simulink model "SF042A_HwAgSnsrls"  (R2013b)
settings: Solver=FixedStepDiscrete  SolverMode=SingleTasking  StartTime=0.0  StopTime=1  FixedStep=0.002  RelTol=1e-3
values from neighbouring files (symbols this model uses):
  ARCHGLBPRM_2MILLISEC_SEC_F32 = DataDict.Constant    [SF042A_HwAgSnsrls_DataDict.m]
  CORRDPINIONAGCON_CNT_U08 = DataDict.Constant    [SF042A_HwAgSnsrls_DataDict.m]
  FCENTROFFSCON_CNT_U08 = DataDict.Constant    [SF042A_HwAgSnsrls_DataDict.m]
  HwAgSnsrlsCorrdPinionAgHwConf = DataDict.Calibration    [SF042A_HwAgSnsrls_DataDict.m]
  HwAgSnsrlsFCentrHwConf = DataDict.Calibration    [SF042A_HwAgSnsrls_DataDict.m]
  HwAgSnsrlsSmotngCoeff = DataDict.Calibration    [SF042A_HwAgSnsrls_DataDict.m]
  HwAgSnsrlsSmotngStepThd = DataDict.Calibration    [SF042A_HwAgSnsrls_DataDict.m]
  HwAgSnsrlsStordPinionConf = DataDict.Calibration    [SF042A_HwAgSnsrls_DataDict.m]
  HwAgSnsrlsStordPinionConfThd = DataDict.Calibration    [SF042A_HwAgSnsrls_DataDict.m]
  HwAgSnsrlsVehDynDifThd = DataDict.Calibration    [SF042A_HwAgSnsrls_DataDict.m]
  HwAgSnsrlsVehDynHwConf = DataDict.Calibration    [SF042A_HwAgSnsrls_DataDict.m]
  HwAgSnsrlsVehDynMotVelThd = DataDict.Calibration    [SF042A_HwAgSnsrls_DataDict.m]
  HwAgSnsrlsVehDynPinionTqThd = DataDict.Calibration    [SF042A_HwAgSnsrls_DataDict.m]
  HwAgSnsrlsVehDynTmr1Thd = DataDict.Calibration    [SF042A_HwAgSnsrls_DataDict.m]
  HwAgSnsrlsVehDynTmr2Thd = DataDict.Calibration    [SF042A_HwAgSnsrls_DataDict.m]
  HwAgSnsrlsVehDynVehSpdThd = DataDict.Calibration    [SF042A_HwAgSnsrls_DataDict.m]
  HwAgSnsrlsVehDynYawRateThd = DataDict.Calibration    [SF042A_HwAgSnsrls_DataDict.m]
  HwAgSnsrlsWhlFrqThd = DataDict.Calibration    [SF042A_HwAgSnsrls_DataDict.m]
  HwAgSnsrlsWhlSpdHwAgCoeff1 = DataDict.Calibration    [SF042A_HwAgSnsrls_DataDict.m]
  HwAgSnsrlsWhlSpdHwAgCoeff2 = DataDict.Calibration    [SF042A_HwAgSnsrls_DataDict.m]
  HwAgSnsrlsWhlSpdHwAgThd = DataDict.Calibration    [SF042A_HwAgSnsrls_DataDict.m]
  HwAgSnsrlsWhlSpdHwConf = DataDict.Calibration    [SF042A_HwAgSnsrls_DataDict.m]
  HwAgSnsrlsWhlSpdRatThd = DataDict.Calibration    [SF042A_HwAgSnsrls_DataDict.m]
  HwAgSnsrlsWhlSpdTmrThd = DataDict.Calibration    [SF042A_HwAgSnsrls_DataDict.m]
  HwAgSnsrlsWhlSpdVehSpdThd = DataDict.Calibration    [SF042A_HwAgSnsrls_DataDict.m]
  LASTPOSNCON_CNT_U08 = DataDict.Constant    [SF042A_HwAgSnsrls_DataDict.m]
  MILLISECTO100MICROSEC_ULS_U32 = DataDict.Constant    [SF042A_HwAgSnsrls_DataDict.m]
  SysGlbPrmSysKineRat = DataDict.ImprtdCal    [SF042A_HwAgSnsrls_DataDict.m]
  SysGlbPrmSysTqRat = DataDict.ImprtdCal    [SF042A_HwAgSnsrls_DataDict.m]
  VEHDYNCON_CNT_U08 = DataDict.Constant    [SF042A_HwAgSnsrls_DataDict.m]
  WHLSPDCON_CNT_U08 = DataDict.Constant    [SF042A_HwAgSnsrls_DataDict.m]
undefined symbols (not defined in the file or in its folder): NtcNr1, SigQlfr1
libraries: NxtrAbslt x11, Fil x8, NxtrLim x4, simulink x3, NxtrNvM x1, FixdToFloat x1
(part 1 of 6)
settings Model: Creator=BZHF94  LastModifiedBy=bzhf94
settings SolverCC: AutoInsertRateTranBlk=on  InsertRTBMode=Always
settings DataIOCC: LimitDataPoints=off  SaveFormat=Structure  ReturnWorkspaceOutputs=on
settings OptimizationCC: BlockReduction=off  InlineParams=on  ZeroExternalMemoryAtStartup=off  ZeroInternalMemoryAtStartup=off  OptimizeModelRefInitCode=on  LifeSpan=1
settings DebuggingCC: SignalInfNanChecking=error  SignalRangeChecking=warning  UnderspecifiedInitializationDetection=Simplified  SolverPrmCheckMsg=error  InheritedTsInSrcMsg=error  DiscreteInheritContinuousMsg=error  SingleTaskRateTransMsg=error  TasksWithSamePriorityMsg=error  SigSpecEnsureSampleTimeMsg=error  CheckMatrixSingularityMsg=error  ParameterUnderflowMsg=error  ParameterPrecisionLossMsg=error  ParameterTunabilityLossMsg=error  FixptConstUnderflowMsg=warning  FixptConstOverflowMsg=warning  VectorMatrixConversionMsg=error  SignalLabelMismatchMsg=error  UnconnectedInputMsg=error  UnconnectedOutputMsg=error  UnconnectedLineMsg=error  SFcnCompatibilityMsg=error  UniqueDataStoreMsg=warning  BusObjectLabelMismatch=error  RootOutportRequireBusObject=error  AssertControl=DisableAll  ModelReferenceIOMsg=error  ModelReferenceVersionMismatchMessage=warning  ModelReferenceIOMismatchMessage=error  ModelReferenceCSMismatchMessage=warning  ModelReferenceDataLoggingMessage=error  StateNameClashWarn=warning  StrictBusMsg=ErrorOnBusTreatedAsVector  NonBusSignalsTreatedAsBus=error  SFUnexpectedBacktrackingDiag=error  SFInvalidInputDataAccessInChartInitDiag=error  SFNoUnconditionalDefaultTransitionDiag=error  SFTransitionOutsideNaturalParentDiag=error  SFUnconditionalTransitionShadowingDiag=error  SFUndirectedBroadcastEventsDiag=error
settings ModelReferenceCC: ModelReferenceNumInstancesAllowed=Single
settings RTWCC: SystemTargetFile=autosar.tlc  GenCodeOnly=on  TemplateMakefile=ert_default_tmf  Description=AUTOSAR  GenerateReport=on  ProcessScript=autosar_make_rtw_hook  LaunchReport=on
settings CodeAppCC: GenerateComments=off  IgnoreCustomStorageClasses=off  CustomSymbolStrType=$N$R$M  CustomSymbolStrBlkIO=$N$M  SimulinkBlockComments=off
settings STFCustomTargetCC: ParMdlRefBuildCompliant=on  CompOptLevelCompliant=on  IncludeMdlTerminateFcn=off  CombineOutputUpdateFcns=on  SuppressErrorStatus=on  ERTFirstTimeCompliant=on  ERTCustomFileBanners=on  SupportNonFinite=off  SupportComplex=off  SupportContinuousTime=off  SupportNonInlinedSFcns=off  MATLABClassNameForMDSCustomization=Simulink.SoftwareTarget.ERTCustomization  AutosarCompliant=on  GRTInterface=off  SystemTargetFile=autosar.tlc
settings ERTTargetCC: CodeReplacementLibrary=ANSI_C  ConcurrentExecutionCompliant=off  IncludeMdlTerminateFcn=off  SuppressErrorStatus=on  SupportNonFinite=off  SupportComplex=off  ModelStepFunctionPrototypeControlCompliant=off  CPPClassGenCompliant=off  AutosarCompliant=on  InlinedParameterPlacement=NonHierarchical  ERTCustomFileTemplate=example_file_process.tlc  EnableUserReplacementTypes=on

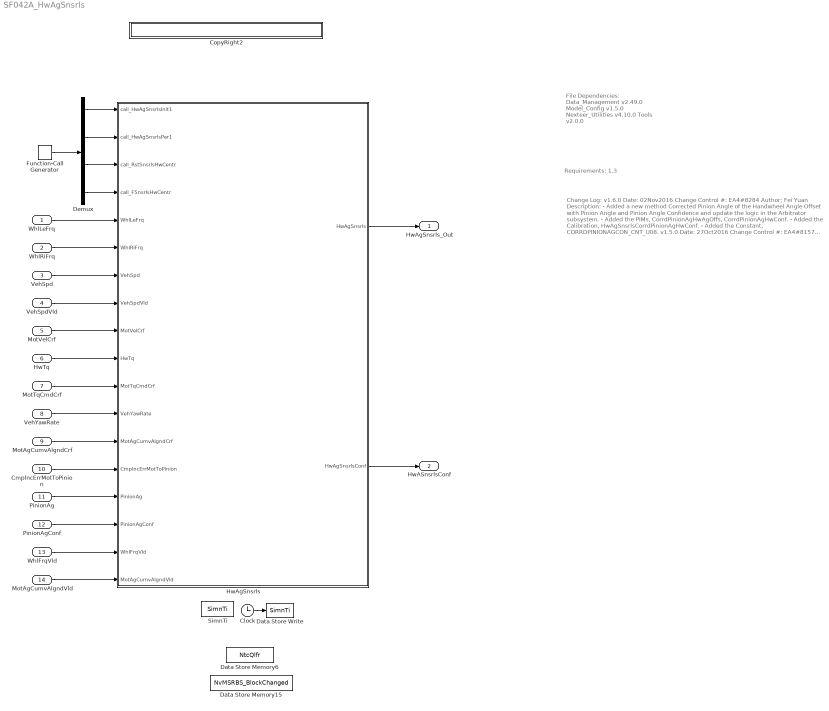
== system SF042A_HwAgSnsrls ==
  note: File Dependencies:
      |
      | Data_Management v2.49.0
      | Model_Config v1.5.0
      | Nexteer_Utilities v4.10.0
      | Tools v2.0.0
  note: Requirements: 1.3
  note: Change Log:
      | v1.6.0
      | Date: 02Nov2016
      | Change Control #: EA4#8284
      | Author: Fei Yuan
      | Description:
      | - Added a new method Corrected Pinion Angle of the Handwheel Angle
      |   Offset with Pinion Angle and Pinion Angle Confidence and update the logic in the
      |   Arbitrator subsystem.
      | - Added the PIMs, CorrdPinionAgHwAgOffs, CorrdPinionAgHwConf.
      | - Added the Calibration, HwAgSnsrlsCorrdPinionAgHwConf.
      | - Added the Constant, CORRDPINIONAGCON_CNT_U08.
      |
      | v1.5.0
      | Date: 27Oct2016
      | Change Control #: EA4#8157
      | Author: Fei Yuan
      | Description:
      | - Change the logic with  (WhlLeFrq - WhlRiFrq)/ (WhlLeFrq + WhlRiFrq) in
      |   WhlSpdRat calculation.
      |
      | v1.4.0
      | Date: 13Oct2016
      | Change Control #: EA4#7996
      | Author: Fei Yuan
      | Description:
      | - Added an input MotAgCumvAlgndVld, two PIMs MotAgOffs and MotAgOffsEna.
      | - Changed the logic in RelPinionAgCalcn subsystem.
      | - Updated the RelPinionAgCalcn to RelHwAgCalcn based on the requirements.
      |
      | v1.3.0
      | Date: 22Sep2016
      | Change Control #: EA4#7682
      | Author: Fei Yuan
      | Description:
      | - Replaced the data type conversion blocks and "Max" blocks with new logic in the
      |   Arbitrator subsystem.
      | - Optimized the "if" logic in the Smoothing subsystem.
      | - Used dHwAgSnsrlsWhlSpdHwConf in the design.
      | - Corrected the unit of HwAgSnsrlsWhlSpdHwConf.
      |
      | v1.2.0
      | Date: 31Aug2016
      | Change Control #: EA4#7070
      | Author: Fei Yuan
      | Description:
      | - Used the previous 4th outcome as the "else" outcome in the Arbitrator subsystem.
      | - Changed the range of PIMs, "WhlSpdHwAgOffs" to [-2440,2440],
      |   "PrevSmotngHwAg" to [-4000,4000].
      | - Removed the PIM, FCentrHwAgEna in the Init1 subsystem and PIM, PrevLrndHwAg,
      |   PrevFildRelHwAg2.
      | - Replaced RELHWAGLOLIM_HWDEG_F32 and RELHWAGHILIM_HWDEG_F32
      |   with HWAGLOLIM_HWDEG_F32 and HWAGHILIM_HWDEG_F32.
      | - Changed MILLISECTOMICROSEC_ULS_U32 to
      |   MILLISECTO100MICROSEC_ULS_U32.
      | - Changed the logic in the Smoothing subsystem.
      | - Changed the HwAgSnsrlsConf.TestTolerance from 0 to 0.004.
      | - Added the PIM, PrevSmotngSt, PrevHwAgOffs, PrevMaxHwConf,
      |   VehDynHwAgOffs.
      | - Added saturation  blocks before writing the value to the NVM StordLstPrm.PinionAg
      |   in the Per1 subsystem.
      | - Replaced the PinionAg with RelHwAg as the input of the Arbitrator subsystem.
      | - Corrected StordLastPrm_SetRamBlockStatus to StordLstPrm_SetRamBlockStatus.
      | - Removed the displays, dHwAgSnsrlsVehDynHwAg, dHwAgSnsrlsWhlSpdHwAg,
      |   dHwAgSnsrlsWhlSpdHwConf.
      | - Changed the logic in the Arbitrator subsystem.
      | - Added links to the design.
      |
      |
      | v1.1.0
      | Date: 01Jul2016
      | CR#: EA4#6474
      | Author: Fei Yuan
      | Description:
      |  - Added "Else" path if WhlFrqVld is false.
      |  - Added "Else" path if no condition is met.
      |  - Added IRVs for StordHwAg and StordHwConf.
      |  - Added SetRamBlockStatus in DataDictionary.
      |  - Changed VehSpdVld datatype to boolean.
      |  - Moved SetRamBlockStatus from Per1 to Init1.
      |
      | v1.0.0
      | Date: 22Jun2016
      | CR#: EA4#6412
      | Author: Fei Yuan
      | Description:
      |  - Initial release in EA4.
  WhlLeFrq : Inport
  WhlRiFrq : Inport  Port=2
  VehSpd : Inport  Port=3
  VehSpdVld : Inport  Port=4
  MotVelCrf : Inport  Port=5
  HwTq : Inport  Port=6
  MotTqCmdCrf : Inport  Port=7
  VehYawRate : Inport  Port=8
  MotAgCumvAlgndCrf : Inport  Port=9
  CmplncErrMotToPinion : Inport  Port=10
  PinionAg : Inport  Port=11
  PinionAgConf : Inport  Port=12
  WhlFrqVld : Inport  Port=13
  MotAgCumvAlgndVld : Inport  Port=14
  Clock : Clock
  CopyRight2 : Subsystem  Description=|  mask(Copyright Information){none=on}
      | Copyright info block.                                               
      |                                                                     
      | Place copyright information at the top of every subsystem in design.
      mask prompts: none "No parameters"
      mask help: Place copyright information at the top of every subsystem in design.
      mask Display:
      | NxtrConf = 'Nexteer Confidential';
      | 
      | sys = bdroot; %handle for the current model ("system")
      | first = get_param(sys,'Created');
      | if(isempty(first))
      |     first = datestr(now,'yyyy');
      | else
      |     first = first(end-3:end);  %year is last four digits
      | end
      | 
      | last = get_param(sys,'LastModifiedDate');
      | if isempty(last)
      |     last = datestr(now,'yyyy');
      | else
      |     last = last(end-3:end);
      | end
      | 
      | if strcmp(first,last)
      |     fprintf('%s -- Copyright %s Nexteer',NxtrConf,first)
      | else
      |     fprintf('%s -- %s%s- %s Nexteer',NxtrConf,char(169),first,last)
      | end
  Data Store Memory15 : DataStoreMemory  DataStoreName=NvMSRBS_BlockChanged  VectorParams1D=off
  Data Store Memory6 : DataStoreMemory  DataStoreName=NtcQlfr  InitialValue=SigQlfr1.SIGQLFR_NORES  OutDataTypeStr=Enum: SigQlfr1
  Data Store Write : DataStoreWrite  DataStoreName=SimnTi
  Demux : Demux
  Function-Call Generator : simulink/Ports & Subsystems/Function-Call Generator  sample_time=0.002  numberOfIterations=1
  HwAgSnsrls : Subsystem
  SimnTi : DataStoreMemory  DataStoreName=SimnTi
  HwAgSnsrls_Out : Outport
  HwASnsrlsConf : Outport  Port=2
  wires:
  Function-Call Generator/1 -> Demux/1
  Demux/4 -> HwAgSnsrls/4(call_FSnsrlsHwCentr)
  Demux/1 -> HwAgSnsrls/1(call_HwAgSnsrlsInit1)
  Demux/2 -> HwAgSnsrls/2(call_HwAgSnsrlsPer1)
  HwAgSnsrls/1(HwAgSnsrls) -> HwAgSnsrls_Out/1
  HwAgSnsrls/2(HwAgSnsrlsConf) -> HwASnsrlsConf/1
  Clock/1 -> Data Store Write/1
  Demux/3 -> HwAgSnsrls/3(call_RstSnsrlsHwCentr)
  WhlLeFrq/1 -> HwAgSnsrls/5(WhlLeFrq)
  WhlRiFrq/1 -> HwAgSnsrls/6(WhlRiFrq)
  PinionAg/1 -> HwAgSnsrls/15(PinionAg)
  CmplncErrMotToPinion/1 -> HwAgSnsrls/14(CmplncErrMotToPinion)
  MotAgCumvAlgndCrf/1 -> HwAgSnsrls/13(MotAgCumvAlgndCrf)
  VehSpdVld/1 -> HwAgSnsrls/8(VehSpdVld)
  MotVelCrf/1 -> HwAgSnsrls/9(MotVelCrf)
  VehYawRate/1 -> HwAgSnsrls/12(VehYawRate)
  HwTq/1 -> HwAgSnsrls/10(HwTq)
  MotTqCmdCrf/1 -> HwAgSnsrls/11(MotTqCmdCrf)
  VehSpd/1 -> HwAgSnsrls/7(VehSpd)
  PinionAgConf/1 -> HwAgSnsrls/16(PinionAgConf)
  WhlFrqVld/1 -> HwAgSnsrls/17(WhlFrqVld)
  MotAgCumvAlgndVld/1 -> HwAgSnsrls/18(MotAgCumvAlgndVld)

== system SF042A_HwAgSnsrls/CopyRight2 ==

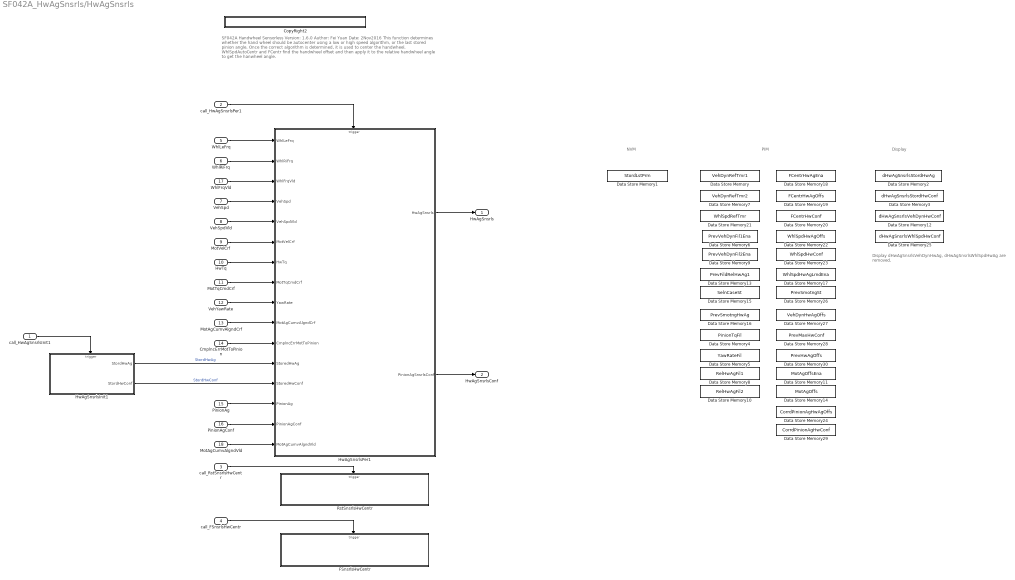
== system SF042A_HwAgSnsrls/HwAgSnsrls ==
  note: Display dHwAgSnsrlsVehDynHwAg, dHwAgSnsrlsWhlSpdHwAg
      | are removed.
  note: SF042A Handwheel Sensorless
      | Version: 1.6.0		Author: Fei Yuan		Date: 2Nov2016
      |
      | This function determines whether the hand wheel should be autocenter using a low or high speed algorithm,
      | or the last stored pinion angle. Once the correct algorithm is determined, it is used to center the handwheel.
      |
      | WhlSpdAutoCentr and FCentr find the handwheel offset and then apply it to the relative handwheel angle to
      |  get the hanwheel angle.
  note: NVM
  note: Display
  note: PIM
  call_HwAgSnsrlsInit1 : Inport
  call_HwAgSnsrlsPer1 : Inport  RequirementInfo={'linktype_rmi_doors' '00012961 (/E-STEER Core/SubSystem Specifications/Application Functions - EA4/SF042A Handwheel Angle Sensorless)' '#SF042A_87' 'true' 'REQ: SF042A_87' '' } %GIDa_10994bec_38d9_4363_acb6_3b85ed334acf  Port=2
  call_RstSnsrlsHwCentr : Inport  Port=3
  call_FSnsrlsHwCentr : Inport  Port=4
  WhlLeFrq : Inport  RequirementInfo={'linktype_rmi_doors' '00012961 (/E-STEER Core/SubSystem Specifications/Application Functions - EA4/SF042A Handwheel Angle Sensorless)' '#SF042A_10' 'true' 'REQ: SF042A_10' '' } %GIDa_ac78d09a_d5a1_45be_aed9_50cdf695eb52  Port=5
  WhlRiFrq : Inport  RequirementInfo={'linktype_rmi_doors' '00012961 (/E-STEER Core/SubSystem Specifications/Application Functions - EA4/SF042A Handwheel Angle Sensorless)' '#SF042A_54' 'true' 'REQ: SF042A_54' '' } %GIDa_9f649e1e_c673_43d0_b21e_596d65fa2f01  Port=6
  VehSpd : Inport  RequirementInfo={'linktype_rmi_doors' '00012961 (/E-STEER Core/SubSystem Specifications/Application Functions - EA4/SF042A Handwheel Angle Sensorless)' '#SF042A_52' 'true' 'REQ: SF042A_52' '' } %GIDa_2d405627_38c6_4c8e_af82_2fc895521a40  Port=7
  VehSpdVld : Inport  RequirementInfo={'linktype_rmi_doors' '00012961 (/E-STEER Core/SubSystem Specifications/Application Functions - EA4/SF042A Handwheel Angle Sensorless)' '#SF042A_51' 'true' 'REQ: SF042A_51' '' } %GIDa_f66125f1_f627_4b6d_9c77_4abd9eee4103  Port=8
  MotVelCrf : Inport  RequirementInfo={'linktype_rmi_doors' '00012961 (/E-STEER Core/SubSystem Specifications/Application Functions - EA4/SF042A Handwheel Angle Sensorless)' '#SF042A_50' 'true' 'REQ: SF042A_50' '' } %GIDa_5a2e065d_6a06_4527_b14a_6c6210358d0c  Port=9
  HwTq : Inport  RequirementInfo={'linktype_rmi_doors' '00012961 (/E-STEER Core/SubSystem Specifications/Application Functions - EA4/SF042A Handwheel Angle Sensorless)' '#SF042A_49' 'true' 'REQ: SF042A_49' '' } %GIDa_0e1bd225_3e57_46aa_ba5f_f2710d75d2e0  Port=10
  MotTqCmdCrf : Inport  RequirementInfo={'linktype_rmi_doors' '00012961 (/E-STEER Core/SubSystem Specifications/Application Functions - EA4/SF042A Handwheel Angle Sensorless)' '#SF042A_48' 'true' 'REQ: SF042A_48' '' } %GIDa_59f05c5a_ba8c_4e2a_876a_661bb90cb7ad  Port=11
  VehYawRate : Inport  RequirementInfo={'linktype_rmi_doors' '00012961 (/E-STEER Core/SubSystem Specifications/Application Functions - EA4/SF042A Handwheel Angle Sensorless)' '#SF042A_47' 'true' 'REQ: SF042A_47' '' } %GIDa_7e6dea3a_393a_451f_b584_a4258df02fc4  Port=12
  MotAgCumvAlgndCrf : Inport  RequirementInfo={'linktype_rmi_doors' '00012961 (/E-STEER Core/SubSystem Specifications/Application Functions - EA4/SF042A Handwheel Angle Sensorless)' '#SF042A_58' 'true' 'REQ: SF042A_58' '' } %GIDa_b20d5ec4_e11b_4d1d_8ee6_c0f83888a87b  Port=13
  CmplncErrMotToPinion : Inport  RequirementInfo={'linktype_rmi_doors' '00012961 (/E-STEER Core/SubSystem Specifications/Application Functions - EA4/SF042A Handwheel Angle Sensorless)' '#SF042A_57' 'true' 'REQ: SF042A_57' '' } %GIDa_e2257f08_1bc5_442f_8487_f2f3dd8c7b68  Port=14
  PinionAg : Inport  RequirementInfo={'linktype_rmi_doors' '00012961 (/E-STEER Core/SubSystem Specifications/Application Functions - EA4/SF042A Handwheel Angle Sensorless)' '#SF042A_56' 'true' 'REQ: SF042A_56' '' } %GIDa_18924965_680c_4e20_b95f_5d9ef85c08bd  Port=15
  PinionAgConf : Inport  RequirementInfo={'linktype_rmi_doors' '00012961 (/E-STEER Core/SubSystem Specifications/Application Functions - EA4/SF042A Handwheel Angle Sensorless)' '#SF042A_55' 'true' 'REQ: SF042A_55' '' } %GIDa_2cd0d863_2f77_4fe6_bae9_0f0f96e25656  Port=16
  WhlFrqVld : Inport  RequirementInfo={'linktype_rmi_doors' '00012961 (/E-STEER Core/SubSystem Specifications/Application Functions - EA4/SF042A Handwheel Angle Sensorless)' '#SF042A_53' 'true' 'REQ: SF042A_53' '' } %GIDa_620c7d14_3b55_4a9d_a417_15032ff26a3c  Port=17
  MotAgCumvAlgndVld : Inport  RequirementInfo={'linktype_rmi_doors' '00012961 (/E-STEER Core/SubSystem Specifications/Application Functions - EA4/SF042A Handwheel Angle Sensorless)' '#SF042A_92' 'true' 'REQ:SF042A_92' '' } %GIDa_d3a0f6d2_bbce_4d6a_8ce9_7a985eaaaca8  Port=18
  CopyRight2 : Subsystem  Description=|  mask(Copyright Information){none=on}
      | Copyright info block.                                               
      |                                                                     
      | Place copyright information at the top of every subsystem in design.
      mask prompts: none "No parameters"
      mask help: Place copyright information at the top of every subsystem in design.
      mask Display:
      | NxtrConf = 'Nexteer Confidential';
      | 
      | sys = bdroot; %handle for the current model ("system")
      | first = get_param(sys,'Created');
      | if(isempty(first))
      |     first = datestr(now,'yyyy');
      | else
      |     first = first(end-3:end);  %year is last four digits
      | end
      | 
      | last = get_param(sys,'LastModifiedDate');
      | if isempty(last)
      |     last = datestr(now,'yyyy');
      | else
      |     last = last(end-3:end);
      | end
      | 
      | if strcmp(first,last)
      |     fprintf('%s -- Copyright %s Nexteer',NxtrConf,first)
      | else
      |     fprintf('%s -- %s%s- %s Nexteer',NxtrConf,char(169),first,last)
      | end
  Data Store Memory : DataStoreMemory  DataStoreName=VehDynRefTmr1  StateMustResolveToSignalObject=on
  Data Store Memory1 : DataStoreMemory  DataStoreName=StordLstPrm  InitialValue=[]  OutDataTypeStr=Bus: StordLstPrmRec1  StateMustResolveToSignalObject=on
  Data Store Memory10 : DataStoreMemory  DataStoreName=RelHwAgFil2  InitialValue=[]  OutDataTypeStr=Bus: FilLpRec1  StateMustResolveToSignalObject=on
  Data Store Memory11 : DataStoreMemory  DataStoreName=MotAgOffsEna  StateMustResolveToSignalObject=on
  Data Store Memory12 : DataStoreMemory  DataStoreName=dHwAgSnsrlsVehDynHwConf  StateMustResolveToSignalObject=on
  Data Store Memory13 : DataStoreMemory  DataStoreName=PrevFildRelHwAg1  StateMustResolveToSignalObject=on
  Data Store Memory14 : DataStoreMemory  DataStoreName=MotAgOffs  StateMustResolveToSignalObject=on
  Data Store Memory15 : DataStoreMemory  DataStoreName=SelnCaseSt  StateMustResolveToSignalObject=on
  Data Store Memory16 : DataStoreMemory  DataStoreName=PrevSmotngHwAg  StateMustResolveToSignalObject=on
  Data Store Memory17 : DataStoreMemory  DataStoreName=WhlSpdHwAgLrndEna  StateMustResolveToSignalObject=on
  Data Store Memory18 : DataStoreMemory  DataStoreName=FCentrHwAgEna  StateMustResolveToSignalObject=on
  Data Store Memory19 : DataStoreMemory  DataStoreName=FCentrHwAgOffs  StateMustResolveToSignalObject=on
  Data Store Memory2 : DataStoreMemory  DataStoreName=dHwAgSnsrlsStordHwAg  StateMustResolveToSignalObject=on
  Data Store Memory20 : DataStoreMemory  DataStoreName=FCentrHwConf  StateMustResolveToSignalObject=on
  Data Store Memory21 : DataStoreMemory  DataStoreName=WhlSpdRefTmr  StateMustResolveToSignalObject=on
  Data Store Memory22 : DataStoreMemory  DataStoreName=WhlSpdHwAgOffs  StateMustResolveToSignalObject=on
  Data Store Memory23 : DataStoreMemory  DataStoreName=WhlSpdHwConf  StateMustResolveToSignalObject=on
  Data Store Memory24 : DataStoreMemory  DataStoreName=CorrdPinionAgHwAgOffs  StateMustResolveToSignalObject=on
  Data Store Memory25 : DataStoreMemory  DataStoreName=dHwAgSnsrlsWhlSpdHwConf  StateMustResolveToSignalObject=on
  Data Store Memory26 : DataStoreMemory  DataStoreName=PrevSmotngSt  StateMustResolveToSignalObject=on
  Data Store Memory27 : DataStoreMemory  DataStoreName=VehDynHwAgOffs  StateMustResolveToSignalObject=on
  Data Store Memory28 : DataStoreMemory  DataStoreName=PrevMaxHwConf  StateMustResolveToSignalObject=on
  Data Store Memory29 : DataStoreMemory  DataStoreName=CorrdPinionAgHwConf  StateMustResolveToSignalObject=on
  Data Store Memory3 : DataStoreMemory  DataStoreName=dHwAgSnsrlsStordHwConf  StateMustResolveToSignalObject=on
  Data Store Memory30 : DataStoreMemory  DataStoreName=PrevHwAgOffs  StateMustResolveToSignalObject=on
  Data Store Memory4 : DataStoreMemory  DataStoreName=PinionTqFil  InitialValue=[]  OutDataTypeStr=Bus: FilLpRec1  StateMustResolveToSignalObject=on
  Data Store Memory5 : DataStoreMemory  DataStoreName=YawRateFil  InitialValue=[]  OutDataTypeStr=Bus: FilLpRec1  StateMustResolveToSignalObject=on
  Data Store Memory6 : DataStoreMemory  DataStoreName=PrevVehDynFil1Ena  StateMustResolveToSignalObject=on
  Data Store Memory7 : DataStoreMemory  DataStoreName=VehDynRefTmr2  StateMustResolveToSignalObject=on
  Data Store Memory8 : DataStoreMemory  DataStoreName=RelHwAgFil1  InitialValue=[]  OutDataTypeStr=Bus: FilLpRec1  StateMustResolveToSignalObject=on
  Data Store Memory9 : DataStoreMemory  DataStoreName=PrevVehDynFil2Ena  StateMustResolveToSignalObject=on
  FSnsrlsHwCentr : Subsystem  RequirementInfo={'linktype_rmi_doors' '00012961 (/E-STEER Core/SubSystem Specifications/Application Functions - EA4/SF042A Handwheel Angle Sensorless)' '#SF042A_61' 'true' 'REQ: SF042A_61' '' } %GIDa_94602c9b_c8a1_4383_ba0b_0fd97e974a1c
  HwAgSnsrlsInit1 : Subsystem
  HwAgSnsrlsPer1 : Subsystem
  RstSnsrlsHwCentr : Subsystem  RequirementInfo={'linktype_rmi_doors' '00012961 (/E-STEER Core/SubSystem Specifications/Application Functions - EA4/SF042A Handwheel Angle Sensorless)' '#SF042A_18' 'true' 'REQ: SF042A_18' '' } %GIDa_ff1cad09_b026_4084_b149_858852ba295c
  HwAgSnsrls : Outport  RequirementInfo={'linktype_rmi_doors' '00012961 (/E-STEER Core/SubSystem Specifications/Application Functions - EA4/SF042A Handwheel Angle Sensorless)' '#SF042A_12' 'true' 'REQ: SF042A_12' '' } %GIDa_5d313ea6_c300_448d_8689_4e05c21cd934
  HwAgSnsrlsConf : Outport  RequirementInfo={'linktype_rmi_doors' '00012961 (/E-STEER Core/SubSystem Specifications/Application Functions - EA4/SF042A Handwheel Angle Sensorless)' '#SF042A_60' 'true' 'REQ: SF042A_60' '' } %GIDa_68a6d026_bfae_4d93_a515_72ebc22a4508  Port=2
  wires:
  VehSpd/1 -> HwAgSnsrlsPer1/4(VehSpd)
  WhlLeFrq/1 -> HwAgSnsrlsPer1/1(WhlLeFrq)
  WhlRiFrq/1 -> HwAgSnsrlsPer1/2(WhlRiFrq)
  WhlFrqVld/1 -> HwAgSnsrlsPer1/3(WhlFrqVld)
  PinionAg/1 -> HwAgSnsrlsPer1/14(PinionAg)
  PinionAgConf/1 -> HwAgSnsrlsPer1/15(PinionAgConf)
  MotVelCrf/1 -> HwAgSnsrlsPer1/6(MotVelCrf)
  MotTqCmdCrf/1 -> HwAgSnsrlsPer1/8(MotTqCmdCrf)
  HwTq/1 -> HwAgSnsrlsPer1/7(HwTq)
  MotAgCumvAlgndCrf/1 -> HwAgSnsrlsPer1/10(MotAgCumvAlgndCrf)
  VehSpdVld/1 -> HwAgSnsrlsPer1/5(VehSpdVld)
  CmplncErrMotToPinion/1 -> HwAgSnsrlsPer1/11(CmplncErrMotToPinion)
  VehYawRate/1 -> HwAgSnsrlsPer1/9(YawRate)
  HwAgSnsrlsPer1/2(PinionAgSnsrlsConf) -> HwAgSnsrlsConf/1
  HwAgSnsrlsPer1/1(HwAgSnsrls) -> HwAgSnsrls/1
  call_HwAgSnsrlsInit1/1 -> HwAgSnsrlsInit1/Trigger
  call_HwAgSnsrlsPer1/1 -> HwAgSnsrlsPer1/Trigger
  HwAgSnsrlsInit1/1(StordHwAg) -> HwAgSnsrlsPer1/12(StoredHwAg)  "StordHwAg"
  call_FSnsrlsHwCentr/1 -> FSnsrlsHwCentr/Trigger
  HwAgSnsrlsInit1/2(StordHwConf) -> HwAgSnsrlsPer1/13(StoredHwConf)  "StordHwConf"
  call_RstSnsrlsHwCentr/1 -> RstSnsrlsHwCentr/Trigger
  MotAgCumvAlgndVld/1 -> HwAgSnsrlsPer1/16(MotAgCumvAlgndVld)

== system SF042A_HwAgSnsrls/HwAgSnsrls/CopyRight2 ==

== system SF042A_HwAgSnsrls/HwAgSnsrls/FSnsrlsHwCentr ==
  function : TriggerPort  TriggerType=function-call
  Constant : Constant  RequirementInfo={'linktype_rmi_doors' '00012961 (/E-STEER Core/SubSystem Specifications/Application Functions - EA4/SF042A Handwheel Angle Sensorless)' '#SF042A_61' 'true' 'REQ: SF042A_61' '' } %GIDa_35363f01_2fa6_4285_8502_0fbb9630c7ae  Value=true  OutDataTypeStr=boolean
      settings: AttributesFormatString=%<OutDataTypeStr>
  CopyRight2 : Subsystem  Description=|  mask(Copyright Information){none=on}
      | Copyright info block.                                               
      |                                                                     
      | Place copyright information at the top of every subsystem in design.
      mask prompts: none "No parameters"
      mask help: Place copyright information at the top of every subsystem in design.
      mask Display:
      | NxtrConf = 'Nexteer Confidential';
      | 
      | sys = bdroot; %handle for the current model ("system")
      | first = get_param(sys,'Created');
      | if(isempty(first))
      |     first = datestr(now,'yyyy');
      | else
      |     first = first(end-3:end);  %year is last four digits
      | end
      | 
      | last = get_param(sys,'LastModifiedDate');
      | if isempty(last)
      |     last = datestr(now,'yyyy');
      | else
      |     last = last(end-3:end);
      | end
      | 
      | if strcmp(first,last)
      |     fprintf('%s -- Copyright %s Nexteer',NxtrConf,first)
      | else
      |     fprintf('%s -- %s%s- %s Nexteer',NxtrConf,char(169),first,last)
      | end
  Data Store Write : DataStoreWrite  RequirementInfo={'linktype_rmi_doors' '00012961 (/E-STEER Core/SubSystem Specifications/Application Functions - EA4/SF042A Handwheel Angle Sensorless)' '#SF042A_61' 'true' 'REQ: SF042A_61' '' } %GIDa_ea1f113f_867c_440b_af3c_3f84bbcf68b4  DataStoreName=FCentrHwAgEna
  wires:
  Constant/1 -> Data Store Write/1

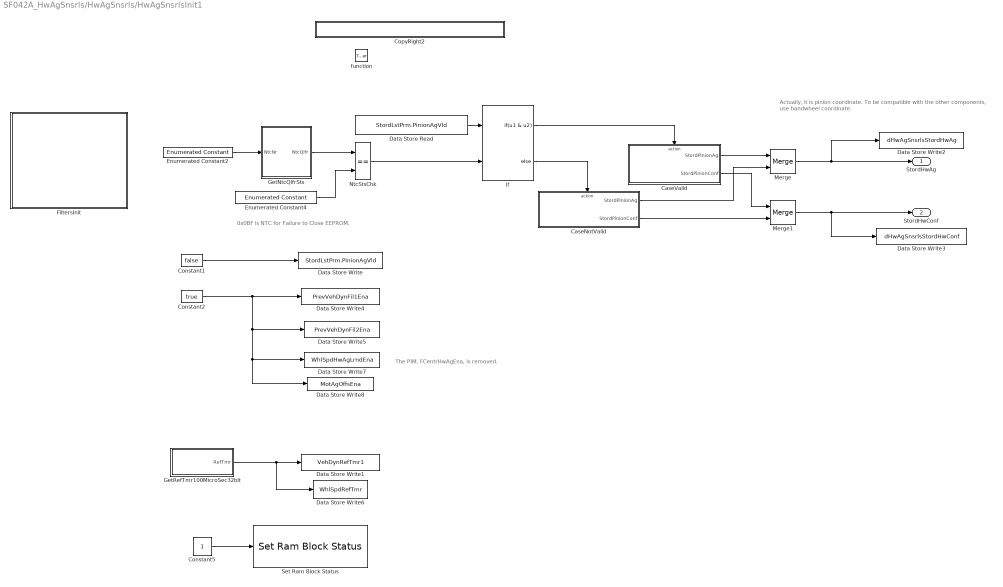
== system SF042A_HwAgSnsrls/HwAgSnsrls/HwAgSnsrlsInit1 ==
  note: The PIM, FCentrHwAgEna, is removed.
  note: Actually, it is pinion coordinate. To be compatible with the other components,
      | use handwheel coordinate.
  note: 0x0BF is NTC for Failure to Close EEPROM.
  function : TriggerPort  TriggerType=function-call
  CaseNotValid : Subsystem  RequirementInfo={'linktype_rmi_doors' '00012961 (/E-STEER Core/SubSystem Specifications/Application Functions - EA4/SF042A Handwheel Angle Sensorless)' '#SF042A_64' 'true' 'REQ: SF042A_64' '' } %GIDa_643d8661_7f2e_44cf_be96_8fcb63329de1  TreatAsAtomicUnit=on
  CaseValid : Subsystem  RequirementInfo={'linktype_rmi_doors' '00012961 (/E-STEER Core/SubSystem Specifications/Application Functions - EA4/SF042A Handwheel Angle Sensorless)' '#SF042A_63' 'true' 'REQ: SF042A_63' '' } %GIDa_d8906579_51af_4ded_af4c_cd59554038e4  TreatAsAtomicUnit=on
  Constant1 : Constant  Value=false  OutDataTypeStr=boolean
      settings: AttributesFormatString=%<OutDataTypeStr>
  Constant2 : Constant  Value=true  OutDataTypeStr=boolean
      settings: AttributesFormatString=%<OutDataTypeStr>
  Constant5 : Constant  RequirementInfo={} %GIDa_7331c101_ab7f_432b_9dd3_936ae6bae64c  OutDataTypeStr=uint8
      settings: AttributesFormatString=%<OutDataTypeStr>
  CopyRight2 : Subsystem  Description=|  mask(Copyright Information){none=on}
      | Copyright info block.                                               
      |                                                                     
      | Place copyright information at the top of every subsystem in design.
      mask prompts: none "No parameters"
      mask help: Place copyright information at the top of every subsystem in design.
      mask Display:
      | NxtrConf = 'Nexteer Confidential';
      | 
      | sys = bdroot; %handle for the current model ("system")
      | first = get_param(sys,'Created');
      | if(isempty(first))
      |     first = datestr(now,'yyyy');
      | else
      |     first = first(end-3:end);  %year is last four digits
      | end
      | 
      | last = get_param(sys,'LastModifiedDate');
      | if isempty(last)
      |     last = datestr(now,'yyyy');
      | else
      |     last = last(end-3:end);
      | end
      | 
      | if strcmp(first,last)
      |     fprintf('%s -- Copyright %s Nexteer',NxtrConf,first)
      | else
      |     fprintf('%s -- %s%s- %s Nexteer',NxtrConf,char(169),first,last)
      | end
  Data Store Read : DataStoreRead  RequirementInfo={'linktype_rmi_doors' '00012961 (/E-STEER Core/SubSystem Specifications/Application Functions - EA4/SF042A Handwheel Angle Sensorless)' '#SF042A_63' 'true' 'REQ: SF042A_63' '' ; 'linktype_rmi_doors' '00012961 (/E-STEER Core/SubSystem Specifications/Application Functions - EA4/SF042A Handwheel Angle Sensorless)' '#SF042A_64' 'true' 'REQ: SF042A_64' '' } %GIDa_c2368b0b_29ed_482a_a3c7_3c6d71fa670b  Priority=1  DataStoreName=StordLstPrm  DataStoreElements=StordLstPrm.PinionAgVld
  Data Store Write : DataStoreWrite  Priority=2  DataStoreName=StordLstPrm  DataStoreElements=StordLstPrm.PinionAgVld
  Data Store Write1 : DataStoreWrite  DataStoreName=VehDynRefTmr1
  Data Store Write2 : DataStoreWrite  DataStoreName=dHwAgSnsrlsStordHwAg
  Data Store Write3 : DataStoreWrite  DataStoreName=dHwAgSnsrlsStordHwConf
  Data Store Write4 : DataStoreWrite  DataStoreName=PrevVehDynFil1Ena
  Data Store Write5 : DataStoreWrite  DataStoreName=PrevVehDynFil2Ena
  Data Store Write6 : DataStoreWrite  DataStoreName=WhlSpdRefTmr
  Data Store Write7 : DataStoreWrite  DataStoreName=WhlSpdHwAgLrndEna
  Data Store Write8 : DataStoreWrite  RequirementInfo={} %GIDa_4447c786_fcaf_45c1_8f5f_f46b218f8a58  DataStoreName=MotAgOffsEna
  Enumerated Constant2 : simulink/Sources/Enumerated Constant  RequirementInfo={'linktype_rmi_doors' '00012961 (/E-STEER Core/SubSystem Specifications/Application Functions - EA4/SF042A Handwheel Angle Sensorless)' '#SF042A_88' 'true' 'REQ: SF042A_88' '' } %GIDa_be7b387a_0e7f_40ff_8eb6_621f0e7404ef  OutDataTypeStr=Enum: NtcNr1  Value=NtcNr1.NTCNR_0X0BF  SampleTime=inf
  Enumerated Constant4 : simulink/Sources/Enumerated Constant  RequirementInfo={'linktype_rmi_doors' '00012961 (/E-STEER Core/SubSystem Specifications/Application Functions - EA4/SF042A Handwheel Angle Sensorless)' '#SF042A_63' 'true' 'REQ: SF042A_63' '' ; 'linktype_rmi_doors' '00012961 (/E-STEER Core/SubSystem Specifications/Application Functions - EA4/SF042A Handwheel Angle Sensorless)' '#SF042A_64' 'true' 'REQ: SF042A_64' '' } %GIDa_dc5f2257_1187_482c_b625_9dc92606ec79  OutDataTypeStr=Enum: SigQlfr1  Value=SigQlfr1.SIGQLFR_PASSD  SampleTime=inf
  FiltersInit : Subsystem
  GetNtcQlfrSts : Subsystem  RequirementInfo={'linktype_rmi_doors' '00012961 (/E-STEER Core/SubSystem Specifications/Application Functions - EA4/SF042A Handwheel Angle Sensorless)' '#SF042A_88' 'true' 'REQ: SF042A_88' '' } %GIDa_1f495d6b_2fae_46a0_b019_8133fb9e0ed3  TreatAsAtomicUnit=on  mask(GetNTC){}
      mask help: GetNTC library block
      settings: RTWSystemCode=Inline
  GetRefTmr100MicroSec32bit : Subsystem  mask(Timer_GRF){}
      mask help: Used to get the reference time in a model.
  If : If  RequirementInfo={'linktype_rmi_doors' '00012961 (/E-STEER Core/SubSystem Specifications/Application Functions - EA4/SF042A Handwheel Angle Sensorless)' '#SF042A_63' 'true' 'REQ: SF042A_63' '' ; 'linktype_rmi_doors' '00012961 (/E-STEER Core/SubSystem Specifications/Application Functions - EA4/SF042A Handwheel Angle Sensorless)' '#SF042A_64' 'true' 'REQ: SF042A_64' '' } %GIDa_8f8077a3_1479_48d8_9186_f4e96cb5f2ad  NumInputs=2  IfExpression=u1 & u2
  Merge : Merge  RequirementInfo={'linktype_rmi_doors' '00012961 (/E-STEER Core/SubSystem Specifications/Application Functions - EA4/SF042A Handwheel Angle Sensorless)' '#SF042A_63' 'true' 'REQ: SF042A_63' '' ; 'linktype_rmi_doors' '00012961 (/E-STEER Core/SubSystem Specifications/Application Functions - EA4/SF042A Handwheel Angle Sensorless)' '#SF042A_64' 'true' 'REQ: SF042A_64' '' } %GIDa_240a166d_69ef_434e_bcca_36284cc46f54
  Merge1 : Merge  RequirementInfo={'linktype_rmi_doors' '00012961 (/E-STEER Core/SubSystem Specifications/Application Functions - EA4/SF042A Handwheel Angle Sensorless)' '#SF042A_63' 'true' 'REQ: SF042A_63' '' ; 'linktype_rmi_doors' '00012961 (/E-STEER Core/SubSystem Specifications/Application Functions - EA4/SF042A Handwheel Angle Sensorless)' '#SF042A_64' 'true' 'REQ: SF042A_64' '' } %GIDa_b7bf3388_b54b_45bf_bff6_b126931c9e85
  NtcStsChk : RelationalOperator  RequirementInfo={'linktype_rmi_doors' '00012961 (/E-STEER Core/SubSystem Specifications/Application Functions - EA4/SF042A Handwheel Angle Sensorless)' '#SF042A_63' 'true' 'REQ: SF042A_63' '' ; 'linktype_rmi_doors' '00012961 (/E-STEER Core/SubSystem Specifications/Application Functions - EA4/SF042A Handwheel Angle Sensorless)' '#SF042A_64' 'true' 'REQ: SF042A_64' '' } %GIDa_0b10b7eb_2e78_417e_af4d_126b5d1d7bcd  Operator===  OutDataTypeStr=boolean
  Set Ram Block Status : NxtrNvM/Set Ram Block Status  RequirementInfo={} %GIDa_829a3bf2_8ab8_4b9c_b14f_259bc887d275  FuncName=Set Ram Block Status  NvMBlockName=StordLstPrm  VoidFuncRtn=on  BlockChanged_DSN=NvMSRBS_BlockChanged  Return_DSN=NvMSRBS_Return
      settings: AttributesFormatString=%<FuncName>
  StordHwAg : Outport
  StordHwConf : Outport  Port=2
  wires:
  Constant5/1 -> Set Ram Block Status/1
  Constant2/1 -> Data Store Write4/1, Data Store Write5/1, Data Store Write8/1, Data Store Write7/1
  CaseNotValid/2(StordPinionConf) -> Merge1/2
  CaseValid/2(StordPinionConf) -> Merge1/1
  CaseValid/1(StordPinionAg) -> Merge/1
  CaseNotValid/1(StordPinionAg) -> Merge/2
  If/2 -> CaseNotValid/Action
  If/1 -> CaseValid/Action
  Data Store Read/1 -> If/1
  NtcStsChk/1 -> If/2
  Enumerated Constant4/1 -> NtcStsChk/2
  Enumerated Constant2/1 -> GetNtcQlfrSts/1(NtcNr)
  GetRefTmr100MicroSec32bit/1(RefTmr) -> Data Store Write1/1, Data Store Write6/1
  Constant1/1 -> Data Store Write/1
  Merge1/1 -> StordHwConf/1, Data Store Write3/1
  Merge/1 -> Data Store Write2/1, StordHwAg/1
  GetNtcQlfrSts/1(NtcQlfr) -> NtcStsChk/1

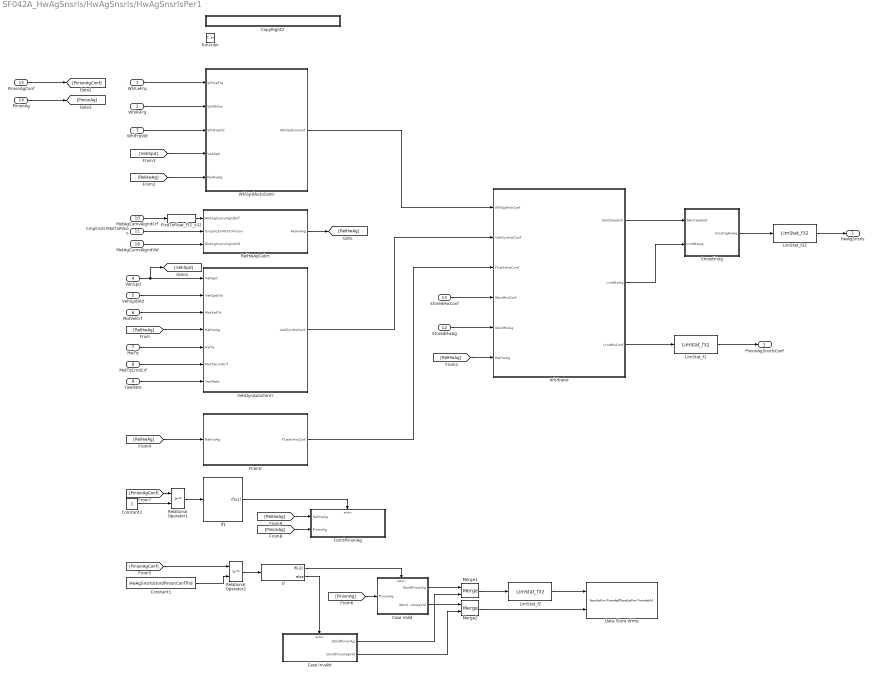
== system SF042A_HwAgSnsrls/HwAgSnsrls/HwAgSnsrlsPer1 ==
  WhlLeFrq : Inport
  WhlRiFrq : Inport  Port=2
  WhlFrqVld : Inport  Port=3
  VehSpd : Inport  Port=4
  VehSpdVld : Inport  Port=5
  MotVelCrf : Inport  Port=6
  HwTq : Inport  Port=7
  MotTqCmdCrf : Inport  Port=8
  YawRate : Inport  Port=9
  MotAgCumvAlgndCrf : Inport  Port=10
  CmplncErrMotToPinion : Inport  Port=11
  StoredHwAg : Inport  Port=12
  StoredHwConf : Inport  Port=13
  PinionAg : Inport  Port=14
  PinionAgConf : Inport  Port=15
  MotAgCumvAlgndVld : Inport  Port=16
  function : TriggerPort  TriggerType=function-call
  Arbitrator : Subsystem
  Case Invalid : Subsystem  RequirementInfo={'linktype_rmi_doors' '00012961 (/E-STEER Core/SubSystem Specifications/Application Functions - EA4/SF042A Handwheel Angle Sensorless)' '#SF042A_72' 'true' 'REQ: SF042A_72' '' } %GIDa_ad86fbd9_b38f_4b8b_a1dc_6633ce75474c  TreatAsAtomicUnit=on
  Case Valid : Subsystem  RequirementInfo={'linktype_rmi_doors' '00012961 (/E-STEER Core/SubSystem Specifications/Application Functions - EA4/SF042A Handwheel Angle Sensorless)' '#SF042A_36' 'true' 'REQ: SF042A_36' '' } %GIDa_ac48a5f0_89a0_4ddd_b42b_d1650f9f3852  TreatAsAtomicUnit=on
  Constant1 : Constant  RequirementInfo={'linktype_rmi_doors' '00012961 (/E-STEER Core/SubSystem Specifications/Application Functions - EA4/SF042A Handwheel Angle Sensorless)' '#SF042A_36' 'true' 'REQ: SF042A_36' '' ; 'linktype_rmi_doors' '00012961 (/E-STEER Core/SubSystem Specifications/Application Functions - EA4/SF042A Handwheel Angle Sensorless)' '#SF042A_72' 'true' 'REQ: SF042A_72' '' } %GIDa_edc5d168_5e8d_4000_ba11_155cb3442b1f  Value=HwAgSnsrlsStordPinionConfThd
  Constant2 : Constant  RequirementInfo="{'linktype_rmi_doors' '00012961 (/E-STEER Core/SubSystem Specifications/Application Functions - EA4/SF042A Handwheel Angle Sensorless)' '#SF042A_36' 'true' 'REQ: SF042A_36' '' ; 'linktype_rmi_doors' '00012961 (/E-STEER Core/SubSystem Specifications/Application Functions - EA4/SF042A Handwheel Angle Sensorless)' '#SF042A_72' 'true' 'REQ: SF042A_72' '' ; 'linktype_rmi_doors' '00012961 (/E-STEER Core/SubSystem Specifications/Application Functions - EA4/SF042A Handwheel Angle Sensorless)' '#SF042A_97' 'true' 'REQ:  SF042A_97' '' ; 'linktype_rmi_doors' '00012961 (/E-STEER Core/SubSystem Specifications/Application Functions - EA4/SF042A Handwheel Angle Sensorless)' '#SF042A_98' 'true' 'REQ:  SF042A_98' '' } %GIDa_d91e313a_8a12_46e4_9b03_ceba33ecba16"  OutDataTypeStr=single
      settings: AttributesFormatString=%<OutDataTypeStr>
  CopyRight2 : Subsystem  Description=|  mask(Copyright Information){none=on}
      | Copyright info block.                                               
      |                                                                     
      | Place copyright information at the top of every subsystem in design.
      mask prompts: none "No parameters"
      mask help: Place copyright information at the top of every subsystem in design.
      mask Display:
      | NxtrConf = 'Nexteer Confidential';
      | 
      | sys = bdroot; %handle for the current model ("system")
      | first = get_param(sys,'Created');
      | if(isempty(first))
      |     first = datestr(now,'yyyy');
      | else
      |     first = first(end-3:end);  %year is last four digits
      | end
      | 
      | last = get_param(sys,'LastModifiedDate');
      | if isempty(last)
      |     last = datestr(now,'yyyy');
      | else
      |     last = last(end-3:end);
      | end
      | 
      | if strcmp(first,last)
      |     fprintf('%s -- Copyright %s Nexteer',NxtrConf,first)
      | else
      |     fprintf('%s -- %s%s- %s Nexteer',NxtrConf,char(169),first,last)
      | end
  CorrdPinionAg : Subsystem  RequirementInfo="{'linktype_rmi_doors' '00012961 (/E-STEER Core/SubSystem Specifications/Application Functions - EA4/SF042A Handwheel Angle Sensorless)' '#SF042A_97' 'true' 'REQ:  SF042A_97' '' ; 'linktype_rmi_doors' '00012961 (/E-STEER Core/SubSystem Specifications/Application Functions - EA4/SF042A Handwheel Angle Sensorless)' '#SF042A_98' 'true' 'REQ:  SF042A_98' '' } %GIDa_06279040_472a_424a_a554_8c95bbc83eb3"  TreatAsAtomicUnit=on
  Data Store Write : DataStoreWrite  DataStoreName=StordLstPrm  DataStoreElements=StordLstPrm.PinionAg#StordLstPrm.PinionAgVld
  FCentr : Subsystem
  FixdToFloat_f32_s32 : FixdToFloat/FixdToFloat_f32_s32  Param1=13
  If : If  RequirementInfo={'linktype_rmi_doors' '00012961 (/E-STEER Core/SubSystem Specifications/Application Functions - EA4/SF042A Handwheel Angle Sensorless)' '#SF042A_36' 'true' 'REQ: SF042A_36' '' ; 'linktype_rmi_doors' '00012961 (/E-STEER Core/SubSystem Specifications/Application Functions - EA4/SF042A Handwheel Angle Sensorless)' '#SF042A_72' 'true' 'REQ: SF042A_72' '' } %GIDa_5071df24_3669_4641_a2d6_25cfa5d6a961  IfExpression=u1
  If1 : If  RequirementInfo="{'linktype_rmi_doors' '00012961 (/E-STEER Core/SubSystem Specifications/Application Functions - EA4/SF042A Handwheel Angle Sensorless)' '#SF042A_97' 'true' 'REQ:  SF042A_97' '' ; 'linktype_rmi_doors' '00012961 (/E-STEER Core/SubSystem Specifications/Application Functions - EA4/SF042A Handwheel Angle Sensorless)' '#SF042A_98' 'true' 'REQ:  SF042A_98' '' } %GIDa_d65c18f0_c1aa_49bc_8b32_e7da5b6e15a2"  IfExpression=u1  ShowElse=off
  LimStat_f1 : NxtrLim/LimStat_f32  LoLim=HWCONFLOLIM_ULS_F32  HiLim=HWCONFHILIM_ULS_F32
      settings: AttributesFormatString=|
      | Low Limit: %<LoLim>
      | High Limit:%<HiLim>
  LimStat_f2 : NxtrLim/LimStat_f32  LoLim=HWAGLOLIM_HWDEG_F32  HiLim=HWAGHILIM_HWDEG_F32
      settings: AttributesFormatString=|
      | Low Limit: %<LoLim>
      | High Limit:%<HiLim>
  LimStat_f32 : NxtrLim/LimStat_f32  LoLim=HWAGLOLIM_HWDEG_F32  HiLim=HWAGHILIM_HWDEG_F32
      settings: AttributesFormatString=|
      | Low Limit: %<LoLim>
      | High Limit:%<HiLim>
  Merge1 : Merge  RequirementInfo={'linktype_rmi_doors' '00012961 (/E-STEER Core/SubSystem Specifications/Application Functions - EA4/SF042A Handwheel Angle Sensorless)' '#SF042A_36' 'true' 'REQ: SF042A_36' '' ; 'linktype_rmi_doors' '00012961 (/E-STEER Core/SubSystem Specifications/Application Functions - EA4/SF042A Handwheel Angle Sensorless)' '#SF042A_72' 'true' 'REQ: SF042A_72' '' } %GIDa_562dd8d7_ee23_42bb_ae13_c87ef4fcc061
  Merge2 : Merge  RequirementInfo={'linktype_rmi_doors' '00012961 (/E-STEER Core/SubSystem Specifications/Application Functions - EA4/SF042A Handwheel Angle Sensorless)' '#SF042A_36' 'true' 'REQ: SF042A_36' '' ; 'linktype_rmi_doors' '00012961 (/E-STEER Core/SubSystem Specifications/Application Functions - EA4/SF042A Handwheel Angle Sensorless)' '#SF042A_72' 'true' 'REQ: SF042A_72' '' } %GIDa_dc859359_5cd1_4500_841a_3e02e6d64341
  RelHwAgCalcn : Subsystem
  Relational Operator1 : RelationalOperator  RequirementInfo="{'linktype_rmi_doors' '00012961 (/E-STEER Core/SubSystem Specifications/Application Functions - EA4/SF042A Handwheel Angle Sensorless)' '#SF042A_36' 'true' 'REQ: SF042A_36' '' ; 'linktype_rmi_doors' '00012961 (/E-STEER Core/SubSystem Specifications/Application Functions - EA4/SF042A Handwheel Angle Sensorless)' '#SF042A_72' 'true' 'REQ: SF042A_72' '' ; 'linktype_rmi_doors' '00012961 (/E-STEER Core/SubSystem Specifications/Application Functions - EA4/SF042A Handwheel Angle Sensorless)' '#SF042A_97' 'true' 'REQ:  SF042A_97' '' ; 'linktype_rmi_doors' '00012961 (/E-STEER Core/SubSystem Specifications/Application Functions - EA4/SF042A Handwheel Angle Sensorless)' '#SF042A_98' 'true' 'REQ:  SF042A_98' '' } %GIDa_8c93600b_cc77_4144_b2a0_5d5d88016206"  OutDataTypeStr=boolean
  Relational Operator2 : RelationalOperator  RequirementInfo={'linktype_rmi_doors' '00012961 (/E-STEER Core/SubSystem Specifications/Application Functions - EA4/SF042A Handwheel Angle Sensorless)' '#SF042A_36' 'true' 'REQ: SF042A_36' '' ; 'linktype_rmi_doors' '00012961 (/E-STEER Core/SubSystem Specifications/Application Functions - EA4/SF042A Handwheel Angle Sensorless)' '#SF042A_72' 'true' 'REQ: SF042A_72' '' } %GIDa_5bd2abee_4e5f_427c_9115_8e7ecb9f4ecc  OutDataTypeStr=boolean
  Smoothing : Subsystem
  VehDynAutoCentr : Subsystem
  WhlSpdAutoCentr : Subsystem
  HwAgSnsrls : Outport
  PinionAgSnsrlsConf : Outport  Port=2
  wires:
  LimStat_f2/1 -> Data Store Write/1
  [RelHwAg] -> FCentr/1(RelHwAg)
  [RelHwAg] -> WhlSpdAutoCentr/5(RelHwAg)
  Merge2/1 -> Data Store Write/2
  Merge1/1 -> LimStat_f2/1
  Case Valid/2(StordPinionAgVld) -> Merge2/1
  Case Invalid/2(StordPinionAgVld) -> Merge2/2
  Case Valid/1(StordPinionAg) -> Merge1/1
  Case Invalid/1(StordPinionAg) -> Merge1/2
  [PinionAg] -> Case Valid/1(PinionAg)
  If/2 -> Case Invalid/Action
  If/1 -> Case Valid/Action
  Relational Operator2/1 -> If/1
  PinionAgConf/1 -> [PinionAgConf]
  Constant1/1 -> Relational Operator2/2
  FixdToFloat_f32_s32/1 -> RelHwAgCalcn/1(MotAgCumvAlgndCrf)
  WhlFrqVld/1 -> WhlSpdAutoCentr/3(WhlFrqVld)
  [VehSpd] -> WhlSpdAutoCentr/4(VehSpd)
  LimStat_f1/1 -> PinionAgSnsrlsConf/1
  LimStat_f32/1 -> HwAgSnsrls/1
  Smoothing/1(SmotngHwAg) -> LimStat_f32/1
  RelHwAgCalcn/1(RelHwAg) -> [RelHwAg]
  CmplncErrMotToPinion/1 -> RelHwAgCalcn/2(CmplncErrMotToPinion)
  MotAgCumvAlgndCrf/1 -> FixdToFloat_f32_s32/1
  WhlRiFrq/1 -> WhlSpdAutoCentr/2(WhlRiFrq)
  WhlLeFrq/1 -> WhlSpdAutoCentr/1(WhlLeFrq)
  YawRate/1 -> VehDynAutoCentr/7(YawRate)
  MotTqCmdCrf/1 -> VehDynAutoCentr/6(MotTqCmdCrf)
  HwTq/1 -> VehDynAutoCentr/5(HwTq)
  [RelHwAg] -> VehDynAutoCentr/4(RelHwAg)
  MotVelCrf/1 -> VehDynAutoCentr/3(MotVelCrf)
  VehSpdVld/1 -> VehDynAutoCentr/2(VehSpdVld)
  VehSpd/1 -> VehDynAutoCentr/1(VehSpd), [VehSpd]
  WhlSpdAutoCentr/1(WhlSpdHwConf) -> Arbitrator/1(WhlSpdHwConf)
  VehDynAutoCentr/1(VehDynHwConf) -> Arbitrator/2(VehDynHwConf)
  StoredHwConf/1 -> Arbitrator/4(StordHwConf)
  FCentr/1(FCentrHwConf) -> Arbitrator/3(FCentrHwConf)
  StoredHwAg/1 -> Arbitrator/5(StordHwAg)
  [RelHwAg] -> Arbitrator/6(RelHwAg)
  Arbitrator/1(SelnCaseSwt) -> Smoothing/1(SelnCaseSwt)
  Arbitrator/2(LrndHwAg) -> Smoothing/2(LrndHwAg)
  Arbitrator/3(LrndHwConf) -> LimStat_f1/1
  MotAgCumvAlgndVld/1 -> RelHwAgCalcn/3(MotAgCumvAlgndVld)
  [PinionAgConf] -> Relational Operator2/1
  PinionAg/1 -> [PinionAg]
  [PinionAgConf] -> Relational Operator1/1
  Constant2/1 -> Relational Operator1/2
  Relational Operator1/1 -> If1/1
  If1/1 -> CorrdPinionAg/Action
  [RelHwAg] -> CorrdPinionAg/1(RelHwAg)
  [PinionAg] -> CorrdPinionAg/2(PinionAg)

== system SF042A_HwAgSnsrls/HwAgSnsrls/RstSnsrlsHwCentr ==
  function : TriggerPort  TriggerType=function-call
  Constant : Constant  RequirementInfo={'linktype_rmi_doors' '00012961 (/E-STEER Core/SubSystem Specifications/Application Functions - EA4/SF042A Handwheel Angle Sensorless)' '#SF042A_18' 'true' 'REQ: SF042A_18' '' } %GIDa_eeb7bc37_1d44_40df_8c9c_f9b041a9d448  Value=false  OutDataTypeStr=boolean
      settings: AttributesFormatString=%<OutDataTypeStr>
  Constant1 : Constant  RequirementInfo={'linktype_rmi_doors' '00012961 (/E-STEER Core/SubSystem Specifications/Application Functions - EA4/SF042A Handwheel Angle Sensorless)' '#SF042A_18' 'true' 'REQ: SF042A_18' '' } %GIDa_1b4c317d_60eb_40f4_a3a7_1140b27fc8c0  Value=0  OutDataTypeStr=single
      settings: AttributesFormatString=%<OutDataTypeStr>
  Constant2 : Constant  RequirementInfo={'linktype_rmi_doors' '00012961 (/E-STEER Core/SubSystem Specifications/Application Functions - EA4/SF042A Handwheel Angle Sensorless)' '#SF042A_18' 'true' 'REQ: SF042A_18' '' } %GIDa_4bf215c1_42aa_4c14_9ad9_171e44161b4a  Value=0  OutDataTypeStr=single
      settings: AttributesFormatString=%<OutDataTypeStr>
  CopyRight2 : Subsystem  Description=|  mask(Copyright Information){none=on}
      | Copyright info block.                                               
      |                                                                     
      | Place copyright information at the top of every subsystem in design.
      mask prompts: none "No parameters"
      mask help: Place copyright information at the top of every subsystem in design.
      mask Display:
      | NxtrConf = 'Nexteer Confidential';
      | 
      | sys = bdroot; %handle for the current model ("system")
      | first = get_param(sys,'Created');
      | if(isempty(first))
      |     first = datestr(now,'yyyy');
      | else
      |     first = first(end-3:end);  %year is last four digits
      | end
      | 
      | last = get_param(sys,'LastModifiedDate');
      | if isempty(last)
      |     last = datestr(now,'yyyy');
      | else
      |     last = last(end-3:end);
      | end
      | 
      | if strcmp(first,last)
      |     fprintf('%s -- Copyright %s Nexteer',NxtrConf,first)
      | else
      |     fprintf('%s -- %s%s- %s Nexteer',NxtrConf,char(169),first,last)
      | end
  Data Store Write : DataStoreWrite  RequirementInfo={'linktype_rmi_doors' '00012961 (/E-STEER Core/SubSystem Specifications/Application Functions - EA4/SF042A Handwheel Angle Sensorless)' '#SF042A_18' 'true' 'REQ: SF042A_18' '' } %GIDa_63c1a626_d62f_4231_8288_3302f49b4f4e  DataStoreName=FCentrHwConf
  Data Store Write2 : DataStoreWrite  RequirementInfo={'linktype_rmi_doors' '00012961 (/E-STEER Core/SubSystem Specifications/Application Functions - EA4/SF042A Handwheel Angle Sensorless)' '#SF042A_18' 'true' 'REQ: SF042A_18' '' } %GIDa_d689b1f2_ef14_435b_8ec1_4eec349c6034  DataStoreName=StordLstPrm  DataStoreElements=StordLstPrm.PinionAg#StordLstPrm.PinionAgVld
  wires:
  Constant2/1 -> Data Store Write/1
  Constant1/1 -> Data Store Write2/1
  Constant/1 -> Data Store Write2/2

== system SF042A_HwAgSnsrls/HwAgSnsrls/FSnsrlsHwCentr/CopyRight2 ==

== system SF042A_HwAgSnsrls/HwAgSnsrls/HwAgSnsrlsInit1/CaseNotValid ==
  Action Port : ActionPort  ActionType=else
  Constant1 : Constant  Value=0  OutDataTypeStr=single
      settings: AttributesFormatString=%<OutDataTypeStr>
  CopyRight2 : Subsystem  Description=|  mask(Copyright Information){none=on}
      | Copyright info block.                                               
      |                                                                     
      | Place copyright information at the top of every subsystem in design.
      mask prompts: none "No parameters"
      mask help: Place copyright information at the top of every subsystem in design.
      mask Display:
      | NxtrConf = 'Nexteer Confidential';
      | 
      | sys = bdroot; %handle for the current model ("system")
      | first = get_param(sys,'Created');
      | if(isempty(first))
      |     first = datestr(now,'yyyy');
      | else
      |     first = first(end-3:end);  %year is last four digits
      | end
      | 
      | last = get_param(sys,'LastModifiedDate');
      | if isempty(last)
      |     last = datestr(now,'yyyy');
      | else
      |     last = last(end-3:end);
      | end
      | 
      | if strcmp(first,last)
      |     fprintf('%s -- Copyright %s Nexteer',NxtrConf,first)
      | else
      |     fprintf('%s -- %s%s- %s Nexteer',NxtrConf,char(169),first,last)
      | end
  StordPinionAg : Outport
  StordPinionConf : Outport  Port=2
  wires:
  Constant1/1 -> StordPinionConf/1, StordPinionAg/1

== system SF042A_HwAgSnsrls/HwAgSnsrls/HwAgSnsrlsInit1/CaseValid ==
  Action Port : ActionPort  ActionType=then
  Constant1 : Constant  Value=HwAgSnsrlsStordPinionConf
  CopyRight2 : Subsystem  Description=|  mask(Copyright Information){none=on}
      | Copyright info block.                                               
      |                                                                     
      | Place copyright information at the top of every subsystem in design.
      mask prompts: none "No parameters"
      mask help: Place copyright information at the top of every subsystem in design.
      mask Display:
      | NxtrConf = 'Nexteer Confidential';
      | 
      | sys = bdroot; %handle for the current model ("system")
      | first = get_param(sys,'Created');
      | if(isempty(first))
      |     first = datestr(now,'yyyy');
      | else
      |     first = first(end-3:end);  %year is last four digits
      | end
      | 
      | last = get_param(sys,'LastModifiedDate');
      | if isempty(last)
      |     last = datestr(now,'yyyy');
      | else
      |     last = last(end-3:end);
      | end
      | 
      | if strcmp(first,last)
      |     fprintf('%s -- Copyright %s Nexteer',NxtrConf,first)
      | else
      |     fprintf('%s -- %s%s- %s Nexteer',NxtrConf,char(169),first,last)
      | end
  Data Store Read1 : DataStoreRead  DataStoreName=StordLstPrm  DataStoreElements=StordLstPrm.PinionAg
  StordPinionAg : Outport
  StordPinionConf : Outport  Port=2
  wires:
  Constant1/1 -> StordPinionConf/1
  Data Store Read1/1 -> StordPinionAg/1

== system SF042A_HwAgSnsrls/HwAgSnsrls/HwAgSnsrlsInit1/CopyRight2 ==
